simulink model "MIP_model"  (R2017a)
settings: Solver=VariableStepAuto  StartTime=0.0  StopTime=10  RelTol=1e-3
settings Model: Creator=ptbrown  LastModifiedBy=ptbrown

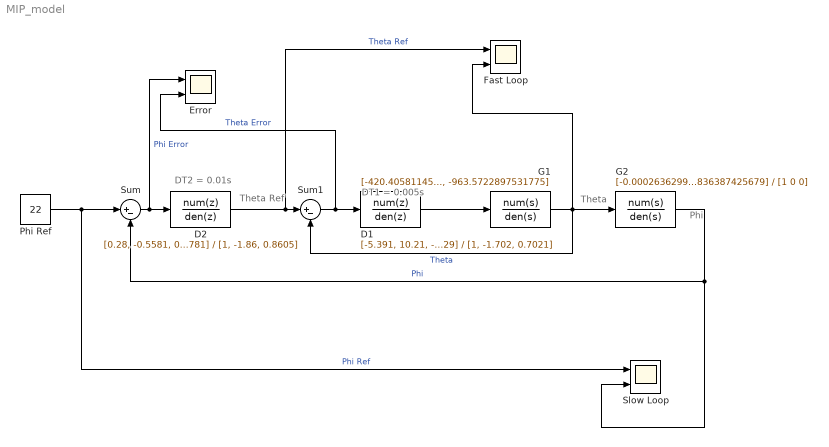
== system MIP_model ==
  note: DT1 = 0.005s
  note: DT2 = 0.01s
  note: Theta Ref
  note: Phi
  note: Theta
  D1 : DiscreteTransferFcn  Numerator=[-5.391, 10.21, -4.829]  Denominator=[1, -1.702, 0.7021]  SampleTime=0.005
  D2 : DiscreteTransferFcn  Numerator=[0.28, -0.5581, 0.2781]  Denominator=[1, -1.86, 0.8605]  SampleTime=0.01
  Error : Scope  NumInputPorts=2
  Fast Loop : Scope  NumInputPorts=2
  G1 : TransferFcn  Numerator=[-420.4058114590155, 0]  Denominator=[1.0000000000000, 12.0975185823100, -88.2402959783804, -963.5722897531775]
  G2 : TransferFcn  Numerator=[-0.0002636299743, 0, 113.3836387425679]  Denominator=[1 0 0]
  Phi Ref : Constant  Value=22
  Slow Loop : Scope  NumInputPorts=2
  Sum : Sum  Inputs=|+-
  Sum1 : Sum  Inputs=|+-
  wires:
  G1/1 -> G2/1, Fast Loop/2, Sum1/2  "Theta"
  Phi Ref/1 -> Sum/1, Slow Loop/1  "Phi Ref"
  Sum/1 -> Error/1, D2/1  "Phi Error"
  D2/1 -> Fast Loop/1, Sum1/1  "Theta Ref"
  Sum1/1 -> Error/2, D1/1  "Theta Error"
  G2/1 -> Sum/2, Slow Loop/2  "Phi"
  D1/1 -> G1/1
